simulink model "Batterymodel_HiL"  (Simulink 7.8)
settings: Solver=FixedStepDiscrete  SolverMode=SingleTasking  StartTime=0.0  StopTime=inf  FixedStep=T_s  RelTol=1e-3
PreLoadFcn:
  | //BatteryParameters;
  | Init_file_Bat
InitFcn:
  | Init_file_Bat;
values from neighbouring files (symbols this model uses):
  C_diff = 5000    [Init_file_Bat.m]
  CellNo = 12    [Init_file_Bat.m]
  ChargeCurrent = 5    [Init_file_Bat.m]
  ChargeSwitch = 1    [Init_file_Bat.m]
  DischargeCurrent = -5    [Init_file_Bat.m]
  n_cells = 12    [Init_file_Bat.m]
  poles_soc = polyfit(SoC_table, OCV_table,4)    [Init_file_Bat.m]
  Q_0 = 36000*ones(1,12)    [Init_file_Bat.m]
  R_ct = 3.2*10^-3    (= 0.0032)    [Init_file_Bat.m]
  R_diff = 4*10^-3    (= 0.004)    [Init_file_Bat.m]
  R_i = 2*10^-3    (= 0.002)    [Init_file_Bat.m]    (also in Kalman_para_int.m = single(0.05))
  SoCinitCells = SoC_init_cells    [Init_file_Bat.m]
  Tcells = T_cells    [Init_file_Bat.m]
  Ts = 10*10^-3    (= 0.01)    [Init_file_Bat.m]
undefined symbols (not defined in the file or in its folder): DiscIntNeverNeededParam, sigbuilder_block
(part 2 of 2)

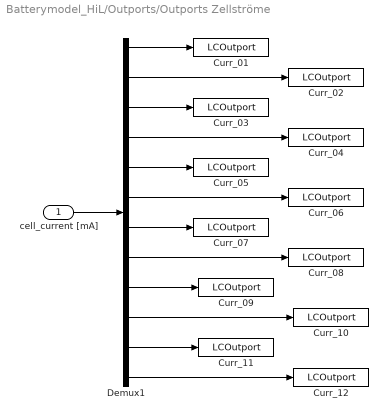
== system Batterymodel_HiL/Outports/Outports Zellströme ==
  cell_current [mA] : Inport
  Curr_01 : S-Function  FunctionName=LCOutport  Parameters=ModelName, OutportID  EnableBusSupport=off  mask(LABCAR Outport){ModelName='Batterymodel_HiL', OutportID=13}
      mask help: This block defines an output of a Simulink model to another module of a LABCAR project
      settings: CopyFcn=set_param( gcb, 'UserData', '####');  OpenFcn=LCOpenFcnCallback
      mask Help:
      | Put this block onto any  hierarchy of the model and connect it to the model.
      | Rename it to any suitable name.
      | Then the corresponding signal is available in the Connection Manager for the wiring to any other module..
  Curr_02 : S-Function  FunctionName=LCOutport  Parameters=ModelName, OutportID  EnableBusSupport=off  mask(LABCAR Outport){ModelName='Batterymodel_HiL', OutportID=14}
      mask help: This block defines an output of a Simulink model to another module of a LABCAR project
      settings: CopyFcn=set_param( gcb, 'UserData', '####');  OpenFcn=LCOpenFcnCallback
      mask Help:
      | Put this block onto any  hierarchy of the model and connect it to the model.
      | Rename it to any suitable name.
      | Then the corresponding signal is available in the Connection Manager for the wiring to any other module..
  Curr_03 : S-Function  FunctionName=LCOutport  Parameters=ModelName, OutportID  EnableBusSupport=off  mask(LABCAR Outport){ModelName='Batterymodel_HiL', OutportID=15}
      mask help: This block defines an output of a Simulink model to another module of a LABCAR project
      settings: CopyFcn=set_param( gcb, 'UserData', '####');  OpenFcn=LCOpenFcnCallback
      mask Help:
      | Put this block onto any  hierarchy of the model and connect it to the model.
      | Rename it to any suitable name.
      | Then the corresponding signal is available in the Connection Manager for the wiring to any other module..
  Curr_04 : S-Function  FunctionName=LCOutport  Parameters=ModelName, OutportID  EnableBusSupport=off  mask(LABCAR Outport){ModelName='Batterymodel_HiL', OutportID=16}
      mask help: This block defines an output of a Simulink model to another module of a LABCAR project
      settings: CopyFcn=set_param( gcb, 'UserData', '####');  OpenFcn=LCOpenFcnCallback
      mask Help:
      | Put this block onto any  hierarchy of the model and connect it to the model.
      | Rename it to any suitable name.
      | Then the corresponding signal is available in the Connection Manager for the wiring to any other module..
  Curr_05 : S-Function  FunctionName=LCOutport  Parameters=ModelName, OutportID  EnableBusSupport=off  mask(LABCAR Outport){ModelName='Batterymodel_HiL', OutportID=17}
      mask help: This block defines an output of a Simulink model to another module of a LABCAR project
      settings: CopyFcn=set_param( gcb, 'UserData', '####');  OpenFcn=LCOpenFcnCallback
      mask Help:
      | Put this block onto any  hierarchy of the model and connect it to the model.
      | Rename it to any suitable name.
      | Then the corresponding signal is available in the Connection Manager for the wiring to any other module..
  Curr_06 : S-Function  FunctionName=LCOutport  Parameters=ModelName, OutportID  EnableBusSupport=off  mask(LABCAR Outport){ModelName='Batterymodel_HiL', OutportID=18}
      mask help: This block defines an output of a Simulink model to another module of a LABCAR project
      settings: CopyFcn=set_param( gcb, 'UserData', '####');  OpenFcn=LCOpenFcnCallback
      mask Help:
      | Put this block onto any  hierarchy of the model and connect it to the model.
      | Rename it to any suitable name.
      | Then the corresponding signal is available in the Connection Manager for the wiring to any other module..
  Curr_07 : S-Function  FunctionName=LCOutport  Parameters=ModelName, OutportID  EnableBusSupport=off  mask(LABCAR Outport){ModelName='Batterymodel_HiL', OutportID=19}
      mask help: This block defines an output of a Simulink model to another module of a LABCAR project
      settings: CopyFcn=set_param( gcb, 'UserData', '####');  OpenFcn=LCOpenFcnCallback
      mask Help:
      | Put this block onto any  hierarchy of the model and connect it to the model.
      | Rename it to any suitable name.
      | Then the corresponding signal is available in the Connection Manager for the wiring to any other module..
  Curr_08 : S-Function  FunctionName=LCOutport  Parameters=ModelName, OutportID  EnableBusSupport=off  mask(LABCAR Outport){ModelName='Batterymodel_HiL', OutportID=20}
      mask help: This block defines an output of a Simulink model to another module of a LABCAR project
      settings: CopyFcn=set_param( gcb, 'UserData', '####');  OpenFcn=LCOpenFcnCallback
      mask Help:
      | Put this block onto any  hierarchy of the model and connect it to the model.
      | Rename it to any suitable name.
      | Then the corresponding signal is available in the Connection Manager for the wiring to any other module..
  Curr_09 : S-Function  FunctionName=LCOutport  Parameters=ModelName, OutportID  EnableBusSupport=off  mask(LABCAR Outport){ModelName='Batterymodel_HiL', OutportID=21}
      mask help: This block defines an output of a Simulink model to another module of a LABCAR project
      settings: CopyFcn=set_param( gcb, 'UserData', '####');  OpenFcn=LCOpenFcnCallback
      mask Help:
      | Put this block onto any  hierarchy of the model and connect it to the model.
      | Rename it to any suitable name.
      | Then the corresponding signal is available in the Connection Manager for the wiring to any other module..
  Curr_10 : S-Function  FunctionName=LCOutport  Parameters=ModelName, OutportID  EnableBusSupport=off  mask(LABCAR Outport){ModelName='Batterymodel_HiL', OutportID=22}
      mask help: This block defines an output of a Simulink model to another module of a LABCAR project
      settings: CopyFcn=set_param( gcb, 'UserData', '####');  OpenFcn=LCOpenFcnCallback
      mask Help:
      | Put this block onto any  hierarchy of the model and connect it to the model.
      | Rename it to any suitable name.
      | Then the corresponding signal is available in the Connection Manager for the wiring to any other module..
  Curr_11 : S-Function  FunctionName=LCOutport  Parameters=ModelName, OutportID  EnableBusSupport=off  mask(LABCAR Outport){ModelName='Batterymodel_HiL', OutportID=23}
      mask help: This block defines an output of a Simulink model to another module of a LABCAR project
      settings: CopyFcn=set_param( gcb, 'UserData', '####');  OpenFcn=LCOpenFcnCallback
      mask Help:
      | Put this block onto any  hierarchy of the model and connect it to the model.
      | Rename it to any suitable name.
      | Then the corresponding signal is available in the Connection Manager for the wiring to any other module..
  Curr_12 : S-Function  FunctionName=LCOutport  Parameters=ModelName, OutportID  EnableBusSupport=off  mask(LABCAR Outport){ModelName='Batterymodel_HiL', OutportID=24}
      mask help: This block defines an output of a Simulink model to another module of a LABCAR project
      settings: CopyFcn=set_param( gcb, 'UserData', '####');  OpenFcn=LCOpenFcnCallback
      mask Help:
      | Put this block onto any  hierarchy of the model and connect it to the model.
      | Rename it to any suitable name.
      | Then the corresponding signal is available in the Connection Manager for the wiring to any other module..
  Demux1 : Demux  Outputs=12
  wires:
  Demux1/2 -> Curr_02/1
  Demux1/1 -> Curr_01/1
  Demux1/3 -> Curr_03/1
  Demux1/4 -> Curr_04/1
  Demux1/6 -> Curr_06/1
  Demux1/8 -> Curr_08/1
  Demux1/7 -> Curr_07/1
  Demux1/5 -> Curr_05/1
  Demux1/10 -> Curr_10/1
  Demux1/12 -> Curr_12/1
  Demux1/9 -> Curr_09/1
  Demux1/11 -> Curr_11/1
  cell_current [mA]/1 -> Demux1/1

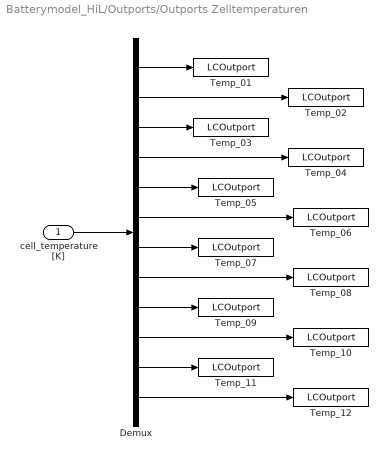
== system Batterymodel_HiL/Outports/Outports Zelltemperaturen ==
  cell_temperature [K] : Inport
  Demux : Demux  Outputs=12
  Temp_01 : S-Function  FunctionName=LCOutport  Parameters=ModelName, OutportID  EnableBusSupport=off  mask(LABCAR Outport){ModelName='Batterymodel_HiL', OutportID=25}
      mask help: This block defines an output of a Simulink model to another module of a LABCAR project
      settings: CopyFcn=set_param( gcb, 'UserData', '####');  OpenFcn=LCOpenFcnCallback
      mask Help:
      | Put this block onto any  hierarchy of the model and connect it to the model.
      | Rename it to any suitable name.
      | Then the corresponding signal is available in the Connection Manager for the wiring to any other module..
  Temp_02 : S-Function  FunctionName=LCOutport  Parameters=ModelName, OutportID  EnableBusSupport=off  mask(LABCAR Outport){ModelName='Batterymodel_HiL', OutportID=26}
      mask help: This block defines an output of a Simulink model to another module of a LABCAR project
      settings: CopyFcn=set_param( gcb, 'UserData', '####');  OpenFcn=LCOpenFcnCallback
      mask Help:
      | Put this block onto any  hierarchy of the model and connect it to the model.
      | Rename it to any suitable name.
      | Then the corresponding signal is available in the Connection Manager for the wiring to any other module..
  Temp_03 : S-Function  FunctionName=LCOutport  Parameters=ModelName, OutportID  EnableBusSupport=off  mask(LABCAR Outport){ModelName='Batterymodel_HiL', OutportID=27}
      mask help: This block defines an output of a Simulink model to another module of a LABCAR project
      settings: CopyFcn=set_param( gcb, 'UserData', '####');  OpenFcn=LCOpenFcnCallback
      mask Help:
      | Put this block onto any  hierarchy of the model and connect it to the model.
      | Rename it to any suitable name.
      | Then the corresponding signal is available in the Connection Manager for the wiring to any other module..
  Temp_04 : S-Function  FunctionName=LCOutport  Parameters=ModelName, OutportID  EnableBusSupport=off  mask(LABCAR Outport){ModelName='Batterymodel_HiL', OutportID=28}
      mask help: This block defines an output of a Simulink model to another module of a LABCAR project
      settings: CopyFcn=set_param( gcb, 'UserData', '####');  OpenFcn=LCOpenFcnCallback
      mask Help:
      | Put this block onto any  hierarchy of the model and connect it to the model.
      | Rename it to any suitable name.
      | Then the corresponding signal is available in the Connection Manager for the wiring to any other module..
  Temp_05 : S-Function  FunctionName=LCOutport  Parameters=ModelName, OutportID  EnableBusSupport=off  mask(LABCAR Outport){ModelName='Batterymodel_HiL', OutportID=29}
      mask help: This block defines an output of a Simulink model to another module of a LABCAR project
      settings: CopyFcn=set_param( gcb, 'UserData', '####');  OpenFcn=LCOpenFcnCallback
      mask Help:
      | Put this block onto any  hierarchy of the model and connect it to the model.
      | Rename it to any suitable name.
      | Then the corresponding signal is available in the Connection Manager for the wiring to any other module..
  Temp_06 : S-Function  FunctionName=LCOutport  Parameters=ModelName, OutportID  EnableBusSupport=off  mask(LABCAR Outport){ModelName='Batterymodel_HiL', OutportID=30}
      mask help: This block defines an output of a Simulink model to another module of a LABCAR project
      settings: CopyFcn=set_param( gcb, 'UserData', '####');  OpenFcn=LCOpenFcnCallback
      mask Help:
      | Put this block onto any  hierarchy of the model and connect it to the model.
      | Rename it to any suitable name.
      | Then the corresponding signal is available in the Connection Manager for the wiring to any other module..
  Temp_07 : S-Function  FunctionName=LCOutport  Parameters=ModelName, OutportID  EnableBusSupport=off  mask(LABCAR Outport){ModelName='Batterymodel_HiL', OutportID=31}
      mask help: This block defines an output of a Simulink model to another module of a LABCAR project
      settings: CopyFcn=set_param( gcb, 'UserData', '####');  OpenFcn=LCOpenFcnCallback
      mask Help:
      | Put this block onto any  hierarchy of the model and connect it to the model.
      | Rename it to any suitable name.
      | Then the corresponding signal is available in the Connection Manager for the wiring to any other module..
  Temp_08 : S-Function  FunctionName=LCOutport  Parameters=ModelName, OutportID  EnableBusSupport=off  mask(LABCAR Outport){ModelName='Batterymodel_HiL', OutportID=32}
      mask help: This block defines an output of a Simulink model to another module of a LABCAR project
      settings: CopyFcn=set_param( gcb, 'UserData', '####');  OpenFcn=LCOpenFcnCallback
      mask Help:
      | Put this block onto any  hierarchy of the model and connect it to the model.
      | Rename it to any suitable name.
      | Then the corresponding signal is available in the Connection Manager for the wiring to any other module..
  Temp_09 : S-Function  FunctionName=LCOutport  Parameters=ModelName, OutportID  EnableBusSupport=off  mask(LABCAR Outport){ModelName='Batterymodel_HiL', OutportID=33}
      mask help: This block defines an output of a Simulink model to another module of a LABCAR project
      settings: CopyFcn=set_param( gcb, 'UserData', '####');  OpenFcn=LCOpenFcnCallback
      mask Help:
      | Put this block onto any  hierarchy of the model and connect it to the model.
      | Rename it to any suitable name.
      | Then the corresponding signal is available in the Connection Manager for the wiring to any other module..
  Temp_10 : S-Function  FunctionName=LCOutport  Parameters=ModelName, OutportID  EnableBusSupport=off  mask(LABCAR Outport){ModelName='Batterymodel_HiL', OutportID=34}
      mask help: This block defines an output of a Simulink model to another module of a LABCAR project
      settings: CopyFcn=set_param( gcb, 'UserData', '####');  OpenFcn=LCOpenFcnCallback
      mask Help:
      | Put this block onto any  hierarchy of the model and connect it to the model.
      | Rename it to any suitable name.
      | Then the corresponding signal is available in the Connection Manager for the wiring to any other module..
  Temp_11 : S-Function  FunctionName=LCOutport  Parameters=ModelName, OutportID  EnableBusSupport=off  mask(LABCAR Outport){ModelName='Batterymodel_HiL', OutportID=35}
      mask help: This block defines an output of a Simulink model to another module of a LABCAR project
      settings: CopyFcn=set_param( gcb, 'UserData', '####');  OpenFcn=LCOpenFcnCallback
      mask Help:
      | Put this block onto any  hierarchy of the model and connect it to the model.
      | Rename it to any suitable name.
      | Then the corresponding signal is available in the Connection Manager for the wiring to any other module..
  Temp_12 : S-Function  FunctionName=LCOutport  Parameters=ModelName, OutportID  EnableBusSupport=off  mask(LABCAR Outport){ModelName='Batterymodel_HiL', OutportID=36}
      mask help: This block defines an output of a Simulink model to another module of a LABCAR project
      settings: CopyFcn=set_param( gcb, 'UserData', '####');  OpenFcn=LCOpenFcnCallback
      mask Help:
      | Put this block onto any  hierarchy of the model and connect it to the model.
      | Rename it to any suitable name.
      | Then the corresponding signal is available in the Connection Manager for the wiring to any other module..
  wires:
  Demux/1 -> Temp_01/1
  Demux/2 -> Temp_02/1
  Demux/3 -> Temp_03/1
  Demux/4 -> Temp_04/1
  Demux/5 -> Temp_05/1
  Demux/6 -> Temp_06/1
  Demux/7 -> Temp_07/1
  Demux/8 -> Temp_08/1
  Demux/10 -> Temp_10/1
  Demux/12 -> Temp_12/1
  Demux/9 -> Temp_09/1
  Demux/11 -> Temp_11/1
  cell_temperature [K]/1 -> Demux/1

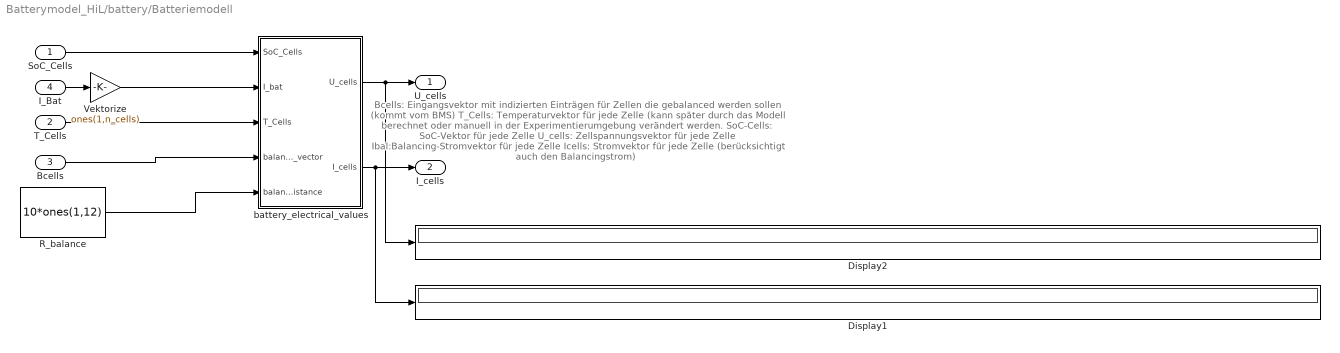
== system Batterymodel_HiL/battery/Batteriemodell ==
  note: Bcells: Eingangsvektor mit indizierten Einträgen
      | für Zellen die gebalanced werden sollen
      | (kommt vom BMS)
      |
      | T_Cells: Temperaturvektor für jede Zelle (kann später
      | durch das Modell berechnet oder manuell in der
      | Experimentierumgebung verändert werden.
      |
      | SoC-Cells: SoC-Vektor für jede Zelle
      |
      | U_cells: Zellspannungsvektor für jede Zelle
      |
      | Ibal:Balancing-Stromvektor für jede Zelle
      |
      | Icells: Stromvektor für jede Zelle (berücksichtigt auch
      | den Balancingstrom)
  SoC_Cells : Inport
  T_Cells : Inport  Port=2
  Bcells : Inport  Port=3
  I_Bat : Inport  Port=4
  Display1 : Display
  Display2 : Display
  R_balance : Constant  Value=10*ones(1,12)
  Vektorize : Gain  Gain=ones(1,n_cells)
  battery_electrical_values : Subsystem
  U_cells : Outport
  I_cells : Outport  Port=2
  wires:
  I_Bat/1 -> Vektorize/1
  SoC_Cells/1 -> battery_electrical_values/1(SoC_Cells)
  T_Cells/1 -> battery_electrical_values/3(T_Cells)
  Vektorize/1 -> battery_electrical_values/2(I_bat)
  Bcells/1 -> battery_electrical_values/4(balance_vector)
  R_balance/1 -> battery_electrical_values/5(balance_resistance)
  battery_electrical_values/1(U_cells) -> U_cells/1, Display2/1
  battery_electrical_values/2(I_cells) -> I_cells/1, Display1/1

== system Batterymodel_HiL/battery/SoC_Cells_Modell ==
  note: Berechnet die individuellen Ladezustände der
      | Zellen ausgehend von einem individuellen
      | Start-Ladezustandswert
  I_cells : Inport
  Init_SoC_Cells : Inport  Port=2
  1/Q_0 : Gain  Gain=1./Q_0
  Add : Sum  Inputs=-+
  Discrete-Time Integrator : DiscreteIntegrator  IntegratorMethod=Integration: Trapezoidal  SampleTime=0.010  ICPrevOutput=DiscIntNeverNeededParam  ICPrevScaledInput=DiscIntNeverNeededParam
  SoC_Cell : Outport
  wires:
  I_cells/1 -> 1/Q_0/1
  Add/1 -> SoC_Cell/1
  Discrete-Time Integrator/1 -> Add/1
  1/Q_0/1 -> Discrete-Time Integrator/1
  Init_SoC_Cells/1 -> Add/2

== system Batterymodel_HiL/displays/Batteirespannung ==
  cell_voltage [V] : Inport
  T1 : Terminator
  T2 : Terminator
  bat_voltage [mV] : Gain  Gain=1000
  sum_bat_voltage [V] : Sum  Inputs=+
  voltage_system : S-Function  FunctionName=LCInport  Parameters=ModelName, InportID, b_useConstant, constValue  EnableBusSupport=off  mask(LABCAR Inport){ModelName='Batterymodel_HiL', InportID=39, b_useConstant=0, constValue=0}
      mask prompts: b_useConstant "Use Constant Value if Online"; constValue "Constant Value"
      mask help: This block gets an input to a Simulink model from another module of a LABCAR project
      settings: CopyFcn=set_param( gcb, 'UserData', '####');  OpenFcn=run LCInportGui
      mask Help:
      | Put this block onto any  hierarchy of the model and connect it to the model.
      | Rename it to any suitable name.
      | Then the corresponding signal is available in the Connection Manager for the wiring to any other module..
  voltage_system [V] : Gain  Gain=1/1000
  voltage_system [mV] : Gain
  wires:
  sum_bat_voltage [V]/1 -> bat_voltage [mV]/1
  bat_voltage [mV]/1 -> T2/1
  cell_voltage [V]/1 -> sum_bat_voltage [V]/1
  voltage_system/1 -> voltage_system [mV]/1
  voltage_system [V]/1 -> T1/1
  voltage_system [mV]/1 -> voltage_system [V]/1

== system Batterymodel_HiL/displays/Batteriestrom ==
  charge current [A] : Inport
  Display : Display
  Display1 : Display
  T1 : Terminator
  T2 : Terminator
  bat_mode_system : S-Function  FunctionName=LCInport  Parameters=ModelName, InportID, b_useConstant, constValue  EnableBusSupport=off  mask(LABCAR Inport){ModelName='Batterymodel_HiL', InportID=40, b_useConstant=0, constValue=0}
      mask prompts: b_useConstant "Use Constant Value if Online"; constValue "Constant Value"
      mask help: This block gets an input to a Simulink model from another module of a LABCAR project
      settings: CopyFcn=set_param( gcb, 'UserData', '####');  OpenFcn=run LCInportGui
      mask Help:
      | Put this block onto any  hierarchy of the model and connect it to the model.
      | Rename it to any suitable name.
      | Then the corresponding signal is available in the Connection Manager for the wiring to any other module..
  charge_current [A] : Gain
  charge_current [mA] : Gain  Gain=1000
  current_system : S-Function  FunctionName=LCInport  Parameters=ModelName, InportID, b_useConstant, constValue  EnableBusSupport=off  mask(LABCAR Inport){ModelName='Batterymodel_HiL', InportID=41, b_useConstant=0, constValue=0}
      mask prompts: b_useConstant "Use Constant Value if Online"; constValue "Constant Value"
      mask help: This block gets an input to a Simulink model from another module of a LABCAR project
      settings: CopyFcn=set_param( gcb, 'UserData', '####');  OpenFcn=run LCInportGui
      mask Help:
      | Put this block onto any  hierarchy of the model and connect it to the model.
      | Rename it to any suitable name.
      | Then the corresponding signal is available in the Connection Manager for the wiring to any other module..
  current_system [A] : Gain  Gain=1/1000
  current_system [mA] : MATLAB Function  TreatAsAtomicUnit=on
  wires:
  charge_current [mA]/1 -> T1/1
  charge current [A]/1 -> charge_current [A]/1, Display1/1
  current_system/1 -> current_system [mA]/1(current_in)
  bat_mode_system/1 -> current_system [mA]/2(bat_mode)
  current_system [mA]/1(current_out) -> current_system [A]/1
  current_system [A]/1 -> T2/1
  charge_current [A]/1 -> charge_current [mA]/1, Display/1

== system Batterymodel_HiL/displays/Vergleich SoC ==
  SoC Modell [%] : Inport
  Cellno : Constant  Value=CellNo
  Data Type Conversion : DataTypeConversion  OutDataTypeStr=single
  SoC : Display
  "SoC Model_% " : Product  Inputs=*/
  SoC1 : Display
  SoC_Kalman : S-Function  FunctionName=LCInport  Parameters=ModelName, InportID, b_useConstant, constValue  EnableBusSupport=off  mask(LABCAR Inport){ModelName='Batterymodel_HiL', InportID=42, b_useConstant=0, constValue=0}
      mask prompts: b_useConstant "Use Constant Value if Online"; constValue "Constant Value"
      mask help: This block gets an input to a Simulink model from another module of a LABCAR project
      settings: CopyFcn=set_param( gcb, 'UserData', '####');  OpenFcn=run LCInportGui
      mask Help:
      | Put this block onto any  hierarchy of the model and connect it to the model.
      | Rename it to any suitable name.
      | Then the corresponding signal is available in the Connection Manager for the wiring to any other module..
  SoC_Kalman_% : Gain  Gain=0.01  OutDataTypeStr=single
  Sum of Elements : Sum  Inputs=+
  T1 : Terminator
  delta SoC : Sum  Inputs=-+
  wires:
  Sum of Elements/1 -> "SoC Model_% "/1
  Cellno/1 -> "SoC Model_% "/2
  "SoC Model_% "/1 -> delta SoC/2, SoC/1
  SoC_Kalman_%/1 -> delta SoC/1
  SoC_Kalman/1 -> Data Type Conversion/1
  Data Type Conversion/1 -> SoC_Kalman_%/1
  SoC Modell [%]/1 -> Sum of Elements/1
  delta SoC/1 -> T1/1, SoC1/1

== system Batterymodel_HiL/Inputs/Charge Profile/virtuel drive cycle ==
  Demux : Demux  Tag=STV Demux  Outputs=1
  FromWs : FromWorkspace  Tag=STV FromWs  VariableName=tuvar  SampleTime=0  SigBuilderData=DataTag40  VnvData=DataTag41
      SigBuilderData=|
      | common.afterFinalStr = 'Extrapolate'
      | common.sampleTime = 0
      | dataSet.timeRange = [0 300]
      | dataSet.name = 'Group 1'
      | sbobj.Groups.Name = 'Group 1'
      | sbobj.Groups.Signals.Name = 'Signal 1'
      | sbobj.Groups.Signals.XData = [0 50 100 110 150 180 200 220 300]
      | sbobj.Groups.Signals.YData = [0 -2 -2.5 0.5 -1 -0.5 -2 1 -1]
      | sbobj.Groups.TimeRange = [0 300]
  Signal 1 : Outport  Tag=STV Outport
  wires:
  Demux/1 -> Signal 1/1
  FromWs/1 -> Demux/1

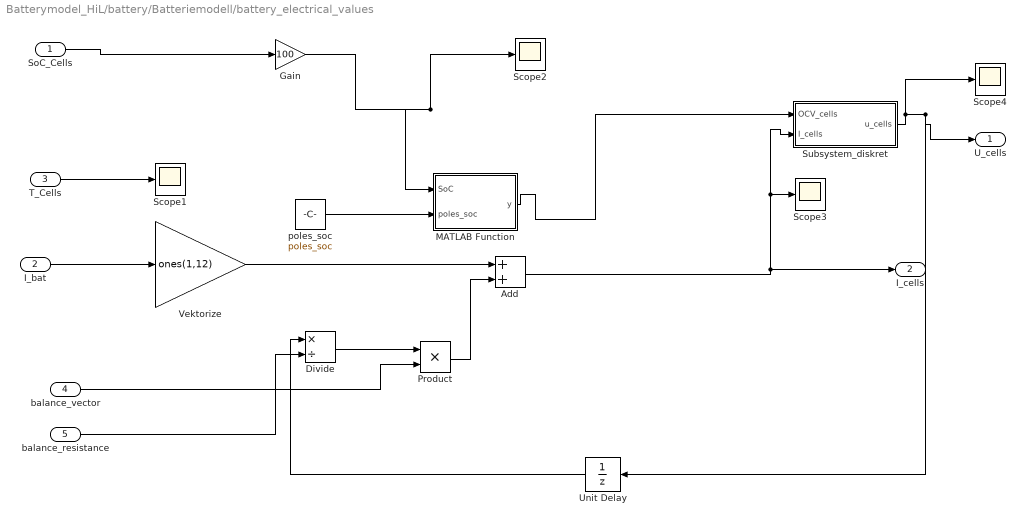
== system Batterymodel_HiL/battery/Batteriemodell/battery_electrical_values ==
  SoC_Cells : Inport
  I_bat : Inport  Port=2
  T_Cells : Inport  Port=3
  balance_vector : Inport  Port=4
  balance_resistance : Inport  Port=5
  " poles_soc" : Constant  Value=poles_soc
  Add : Sum
  Divide : Product  Inputs=*/
  Gain : Gain  Gain=100
  MATLAB Function : MATLAB Function  TreatAsAtomicUnit=on
  Product : Product  RndMeth=Zero
  Scope{1..4} (4 alike) : Scope
      Scope1 settings: YMin=41  YMax=50
      Scope2 settings: YMin=41  YMax=50  SaveName=ScopeData5
      Scope3 settings: SaveName=ScopeData6
      Scope4 settings: YMin=2.6  YMax=3.45  SaveName=ScopeData10
  Subsystem_diskret : Subsystem
  Unit Delay : UnitDelay  SampleTime=-1
  Vektorize : Gain  Gain=ones(1,12)
  U_cells : Outport
  I_cells : Outport  Port=2
  wires:
  SoC_Cells/1 -> Gain/1
  Subsystem_diskret/1(u_cells) -> Scope4/1, U_cells/1, Unit Delay/1
  I_bat/1 -> Vektorize/1
  Gain/1 -> Scope2/1, MATLAB Function/1(SoC)
  MATLAB Function/1(y) -> Subsystem_diskret/1(OCV_cells)
  " poles_soc"/1 -> MATLAB Function/2(poles_soc)
  balance_vector/1 -> Product/2
  Product/1 -> Add/2
  balance_resistance/1 -> Divide/2
  Vektorize/1 -> Add/1
  Add/1 -> I_cells/1, Subsystem_diskret/2(I_cells), Scope3/1
  Divide/1 -> Product/1
  T_Cells/1 -> Scope1/1
  Unit Delay/1 -> Divide/1

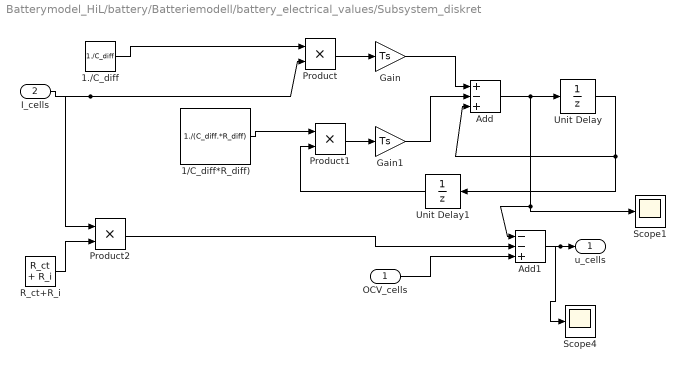
== system Batterymodel_HiL/battery/Batteriemodell/battery_electrical_values/Subsystem_diskret ==
  OCV_cells : Inport
  I_cells : Inport  Port=2
  1./C_diff : Constant  Value=1./C_diff
  1/C_diff*R_diff) : Constant  Value=1./(C_diff.*R_diff)
  Add : Sum  Inputs=+-+
  Add1 : Sum  Inputs=--+
  Gain : Gain  Gain=Ts
  Gain1 : Gain  Gain=Ts
  Product : Product  RndMeth=Zero
  Product1 : Product  RndMeth=Zero
  Product2 : Product  RndMeth=Zero
  R_ct+R_i : Constant  Value=R_ct + R_i
  Scope1 : Scope
      settings: TimeRange=4500  YMin=3.25  YMax=3.55  SaveName=ScopeData7
  Scope4 : Scope
      settings: TimeRange=4500  YMin=3.25  YMax=3.55  SaveName=ScopeData11
  Unit Delay : UnitDelay  SampleTime=-1
  Unit Delay1 : UnitDelay  SampleTime=-1
  u_cells : Outport
  wires:
  1./C_diff/1 -> Product/1
  I_cells/1 -> Product/2, Product2/1
  Gain/1 -> Add/1
  Add/1 -> Unit Delay/1, Add1/1, Scope1/1
  1/C_diff*R_diff)/1 -> Product1/1
  Unit Delay/1 -> Add/3, Unit Delay1/1
  Product1/1 -> Gain1/1
  Add1/1 -> u_cells/1, Scope4/1
  Product2/1 -> Add1/2
  OCV_cells/1 -> Add1/3
  R_ct+R_i/1 -> Product2/2
  Product/1 -> Gain/1
  Gain1/1 -> Add/2
  Unit Delay1/1 -> Product1/2

== matlab function displays/Batteriestrom/current_system [mA] ==
  data: current_out output double; current_in input double; bat_mode input double
function current_out  = fcn(current_in, bat_mode)

if (bat_mode == 0)
    current = current_in;
else
    current = current_in*(-1);
end

%Ausgabe
current_out = current;

== matlab function Outports/Embedded MATLAB Function ==
  data: current input double; bat_modus output double
function bat_modus = fcn(current)

if current > 0
    bat_modus = 0;
else
    bat_modus = 1;
end

== matlab function battery/Batteriemodell/battery_electrical_values/MATLAB Function ==
  data: SoC input double; y output double; poles_soc input double
function y = fcn(SoC, poles_soc)
y= polyval(poles_soc, SoC);
